simulink model "provaTuningRadio"  (R2023b)
settings: Solver=FixedStepAuto  StartTime=0.0  StopTime=2e5  FixedStep=10  RelTol=1e-3
undefined symbols (not defined in the file or in its folder): Radio
libraries: sensors_subsystems x3, simulink x1
settings Model: DataDictionary=SimulationDict.sldd  SimulationMode=accelerator  Creator=brent  LastModifiedBy=brent

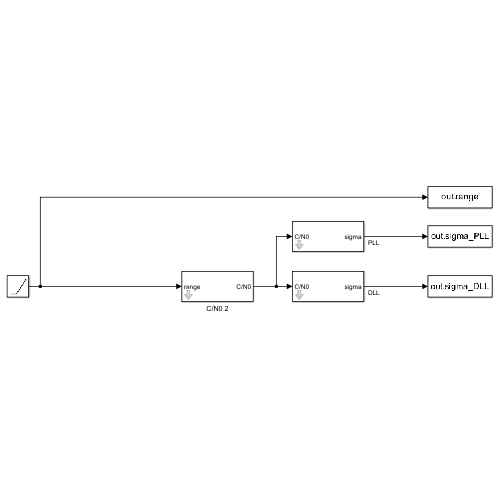
[thumbnail: Simulink's stored preview of the top-level diagram]
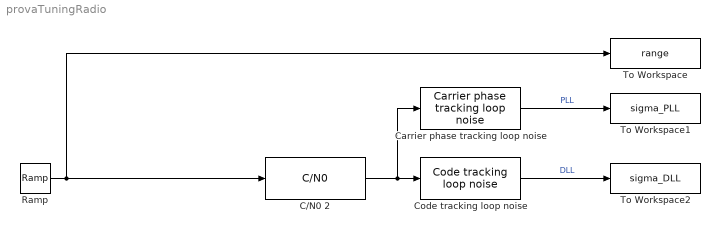
== system provaTuningRadio ==
  C/N0 2 : sensors_subsystems/C//N0  lambda=Radio.lambda.value  Pt=Radio.Tx.P.value  Gt=Radio.Tx.gain.value  Gr=Radio.Rx.gain.value  N0=Radio.N0.value  L_rx=Radio.Rx.losses.value
      settings: SourceProductName=Sensors library
  Carrier phase tracking loop noise : sensors_subsystems/Carrier phase tracking loop noise  Bn=Radio.Phase.Bn.value  T=Radio.Phase.T.value  lambda=Radio.lambda.value
      settings: SourceProductName=Sensors library
  Code tracking loop noise : sensors_subsystems/Code tracking loop noise  Bn=Radio.PN.Bn.value  D=Radio.PN.D.value  T=Radio.PN.T.value  Tc=Radio.PN.Tc.value  Bfe=Radio.PN.Bfe.value  lambda=Radio.PN.lambda_c.value
      settings: SourceProductName=Sensors library
  Ramp : simulink/Sources/Ramp  slope=1e3  start=0  InitialOutput=6e5
  To Workspace : ToWorkspace  VariableName=range  SampleTime=-1
      settings: Save2DSignal=2-D array (concatenate along first dimension)
  To Workspace1 : ToWorkspace  VariableName=sigma_PLL  SampleTime=-1
      settings: Save2DSignal=2-D array (concatenate along first dimension)
  To Workspace2 : ToWorkspace  VariableName=sigma_DLL  SampleTime=-1
      settings: Save2DSignal=2-D array (concatenate along first dimension)
  wires:
  C/N0 2/1 -> Carrier phase tracking loop noise/1, Code tracking loop noise/1
  Carrier phase tracking loop noise/1 -> To Workspace1/1  "PLL"
  Code tracking loop noise/1 -> To Workspace2/1  "DLL"
  Ramp/1 -> To Workspace/1, C/N0 2/1
